simulink model "uklad1"  (R2023a)
settings: Solver=VariableStepAuto  StartTime=0.0  StopTime=50  RelTol=1e-3
undefined symbols (not defined in the file): k, T, Tp
settings Model: Creator=jpawl  LastModifiedBy=jpawl

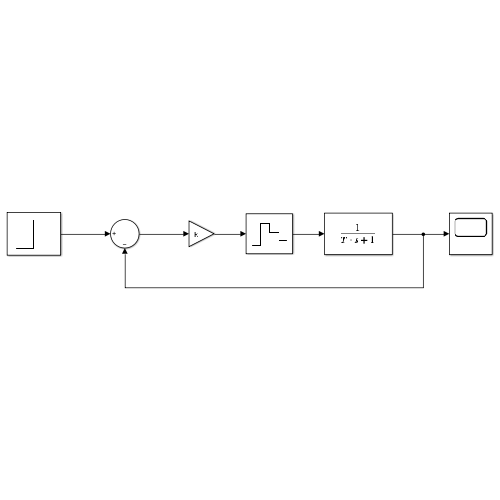
[thumbnail: Simulink's stored preview of the top-level diagram]
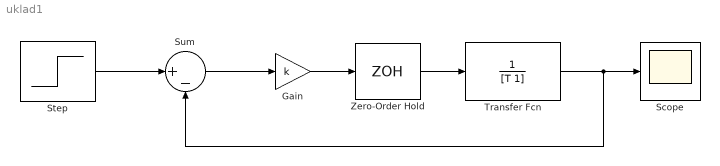
== system uklad1 ==
  Gain : Gain  Gain=k
  Scope : Scope
  Step : Step  SampleTime=Tp
  Sum : Sum  Inputs=|+-
  Transfer Fcn : TransferFcn  Denominator=[T 1]
  Zero-Order Hold : ZeroOrderHold  SampleTime=Tp
  wires:
  Step/1 -> Sum/1
  Sum/1 -> Gain/1
  Gain/1 -> Zero-Order Hold/1
  Zero-Order Hold/1 -> Transfer Fcn/1
  Transfer Fcn/1 -> Sum/2, Scope/1
